simulink model "FORK"  (R2013b)
settings: Solver=ode45  StartTime=0.0  StopTime=2  RelTol=1e-3
libraries: powerlib x36, powerlib_meascontrol x6, powerlib_extras x3
settings Model: Creator=Yugal  LastModifiedBy=internship

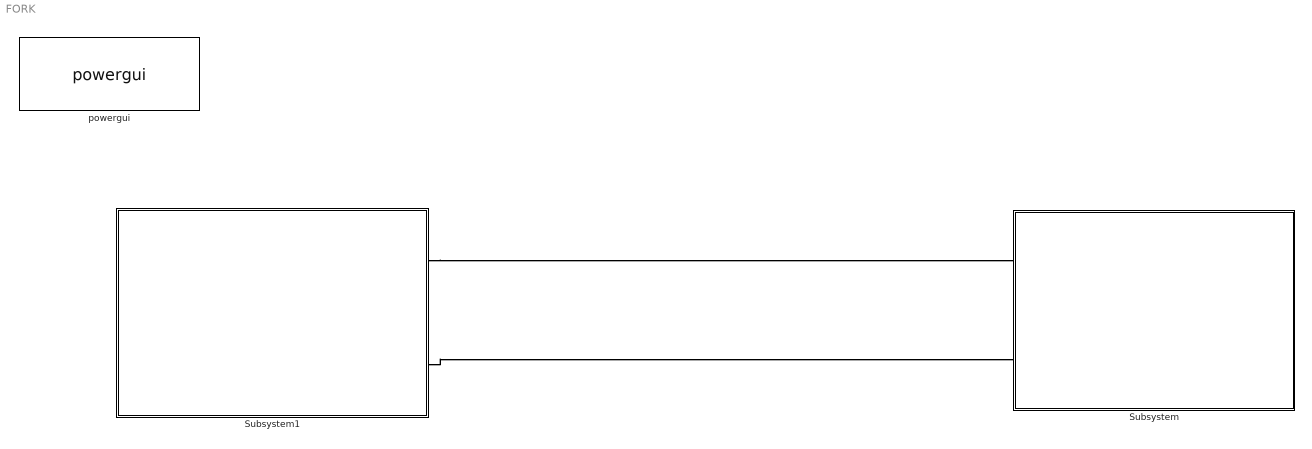
== system FORK ==
  Subsystem : Subsystem
  Subsystem1 : Subsystem
  powergui : powerlib/powergui  Priority=1  SimulationMode=Discrete  SolverType=Tustin  SampleTime=10e-6  frequency=60  SPID=off  DisableSnubberDevices=off  DisableRonSwitches=off  DisableVfSwitches=off  SwTol=0  Interpol=off  DisplayEquations=off  frequencyindice=50  Pbase=100e6  ErrMax=1e-4  Iterations=50  UnitsV=kV  UnitsW=MW  FunctionMessages=off  echomessages=off  HookPort=off  EnableUseOfTLC=off  x0status=blocks  RestoreLinks=warning  ResistiveCurrentMeasurement=off  Frange=[0:2:500]  Ylog=off  Xlog=on  ShowGrid=off  save=off  variable=ZData  structure=Ia  ZoomFFT=on  StartTime=1.5  cycles=2  DisplayStyle=1  fundamental=50  FreqAxis=on  MaxFrequency=1000  frequencyindicesteady=1  RmsSteady=1  display=off  Ts=100  methode=off
  connections:
  Subsystem1/RConn1 -- Subsystem/LConn1
  Subsystem1/RConn2 -- Subsystem/LConn2

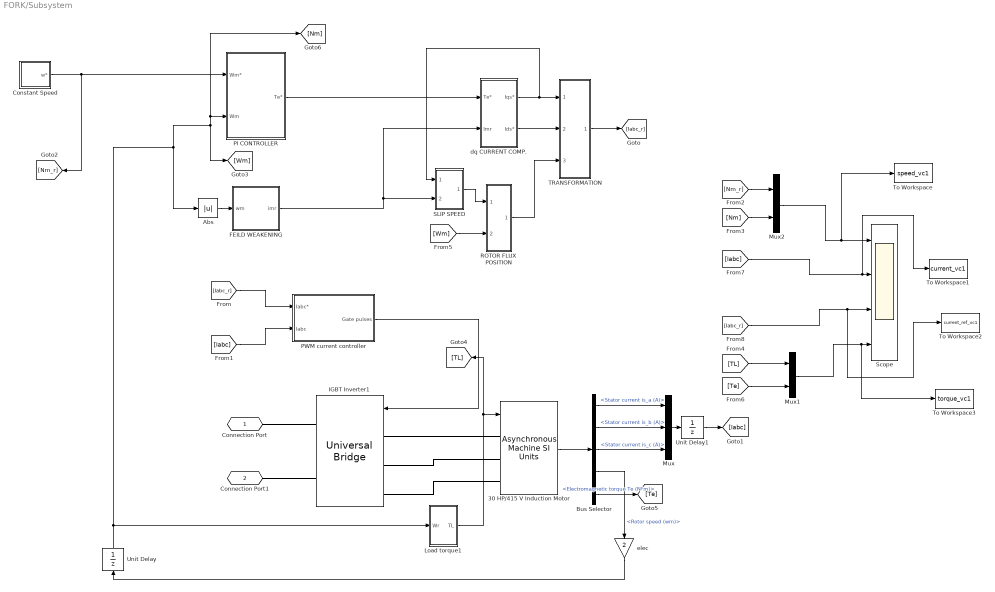
== system FORK/Subsystem ==
  30 HP/415 V Induction Motor : powerlib/Machines/Asynchronous Machine SI Units  PresetModel=No  MechanicalLoad=Torque Tm  ShowDetailedParameters=on  RotorType=Squirrel-cage  ReferenceFrame=Rotor  NominalParameters=[30*746 415 50]  Stator=[0.251 0.001397]  Rotor=[0.249 0.001397]  Cage1=[ 0.022 0.226/377]  Cage2=[ 0.022 0.226/377]  Lm=0.0416  Mechanical=[0.305 0 2 ]  PolePairs=2  InitialConditions=[1 0 0 0 0 0 0 0]  Units=SI  LoadFlowParameters=1492000  SimulateSaturation=off  Saturation=[14.03593122, 27.81365428, 53.79336849, 72.68890987, 97.98006896, 148.6815601, 215.7428561, 302.9841135, 420.4778367 ; 230, 322, 414, 460, 506, 552, 598, 644, 690]  TsPowergui=0  TsBlock=-1  IterativeModel=Trapezoidal non iterative  Pmec=0
  Abs : Abs  SaturateOnIntegerOverflow=on
  Bus Selector : BusSelector  OutputSignals=Stator measurements.Stator current is_a (A),Stator measurements.Stator current is_b (A),Stator measurements.Stator current is_c (A),Mechanical.Rotor speed (wm),Mechanical.Electromagnetic torque Te (N*m)
  Constant Speed : Subsystem
  FEILD WEAKENING : MATLAB Function  TreatAsAtomicUnit=on
  IGBT Inverter1 : powerlib/Power Electronics/Universal Bridge  Arms=3  SnubberResistance=1e5  SnubberCapacitance=inf  Device=MOSFET / Diodes  Ron=1e-3  Lon=0  ForwardVoltages="[  0  0  ]"  ForwardVoltage=0  GTOparameters=[ 10e-6 , 20e-6 ]  IGBTparameters=[ 1e-6 , 2e-6 ]  Measurements=None  Measurements_2=None  converterType=Rectifier
  Load torque1 : Subsystem
  Mux : Mux  Inputs=3
  Mux1 : Mux  Inputs=2
  Mux2 : Mux  Inputs=2
  PI CONTROLLER : Subsystem  mask{Kp=90, Ki=2.6, Ts=100e-6, Lim=300}
      mask prompts: Ts "Sampling Time Ts (sec)"; Lim "Ref Torque limit(N-m)"
  PWM current controller : Subsystem
  ROTOR FLUX POSITION : Subsystem
  SLIP SPEED : Subsystem
  Scope : Scope  NumInputPorts=4
      settings: TickLabels=on  TimeRange=4.5  YMin=249.989~-25~-22.5~-11  YMax=250.008~25~22.5~7  MaxDataPoints=1000  Decimation=10
  TRANSFORMATION : Subsystem
  To Workspace : ToWorkspace  VariableName=speed_vc1  SampleTime=100e-6  SaveFormat=Structure With Time
  To Workspace1 : ToWorkspace  VariableName=current_vc1  SampleTime=100e-6  SaveFormat=Structure With Time
  To Workspace2 : ToWorkspace  VariableName=current_ref_vc1  SampleTime=100e-6  SaveFormat=Structure With Time
  To Workspace3 : ToWorkspace  VariableName=torque_vc1  SampleTime=100e-6  SaveFormat=Structure With Time
  Unit Delay : UnitDelay  SampleTime=100e-6
  Unit Delay1 : UnitDelay  SampleTime=10e-6
  dq CURRENT COMP. : Subsystem
  elec : Gain  Gain=2
  Connection Port : PMIOPort  Port=1  Side=Left
  Connection Port1 : PMIOPort  Port=2  Side=Left
  wires:
  PWM current controller/1(Gate pulses) -> IGBT Inverter1/1
  Load torque1/1(TL) -> [TL], 30 HP/415 V Induction Motor/1
  30 HP/415 V Induction Motor/1 -> Bus Selector/1
  Bus Selector/3 -> Mux/3  "<Stator current is_c (A)>"
  Bus Selector/2 -> Mux/2  "<Stator current is_b (A)>"
  Bus Selector/1 -> Mux/1  "<Stator current is_a (A)>"
  [Iabc] -> PWM current controller/2(Iabc)
  [Iabc_r] -> PWM current controller/1(Iabc*)
  Abs/1 -> FEILD WEAKENING/1(wm)
  dq CURRENT COMP./2(Ids*) -> TRANSFORMATION/2(Ids*)
  dq CURRENT COMP./1(Iqs*) -> SLIP SPEED/1(Iqs*), TRANSFORMATION/1(Iqs*)
  PI CONTROLLER/1(Te*) -> dq CURRENT COMP./1(Te*)
  FEILD WEAKENING/1(imr) -> SLIP SPEED/2(Imr*), dq CURRENT COMP./2(Imr)
  SLIP SPEED/1(Wsl) -> ROTOR FLUX POSITION/1("Wsl\t")
  ROTOR FLUX POSITION/1(theta) -> TRANSFORMATION/3(theta)
  [Wm] -> ROTOR FLUX POSITION/2(Wm)
  TRANSFORMATION/1(Iabc*) -> [Iabc_r]
  Bus Selector/5 -> [Te]  "<Electromagnetic torque Te (N*m)>"
  [Te] -> Mux1/2
  [TL] -> Mux1/1
  Bus Selector/4 -> elec/1  "<Rotor speed (wm)>"
  Mux1/1 -> To Workspace3/1, Scope/4
  [Nm_r] -> Mux2/1
  [Nm] -> Mux2/2
  Mux2/1 -> To Workspace/1, Scope/1
  [Iabc] -> To Workspace1/1, Scope/2
  Constant Speed/1(w*) -> PI CONTROLLER/1(Wm*), [Nm_r]
  [Iabc_r] -> To Workspace2/1, Scope/3
  Mux/1 -> Unit Delay1/1
  Unit Delay1/1 -> [Iabc]
  elec/1 -> Unit Delay/1
  Unit Delay/1 -> Load torque1/1(Wr), [Nm], PI CONTROLLER/2(Wm), [Wm], Abs/1
  connections:
  30 HP/415 V Induction Motor/LConn1 -- IGBT Inverter1/LConn1
  30 HP/415 V Induction Motor/LConn3 -- IGBT Inverter1/LConn3
  30 HP/415 V Induction Motor/LConn2 -- IGBT Inverter1/LConn2
  Connection Port/RConn1 -- IGBT Inverter1/RConn1
  Connection Port1/RConn1 -- IGBT Inverter1/RConn2

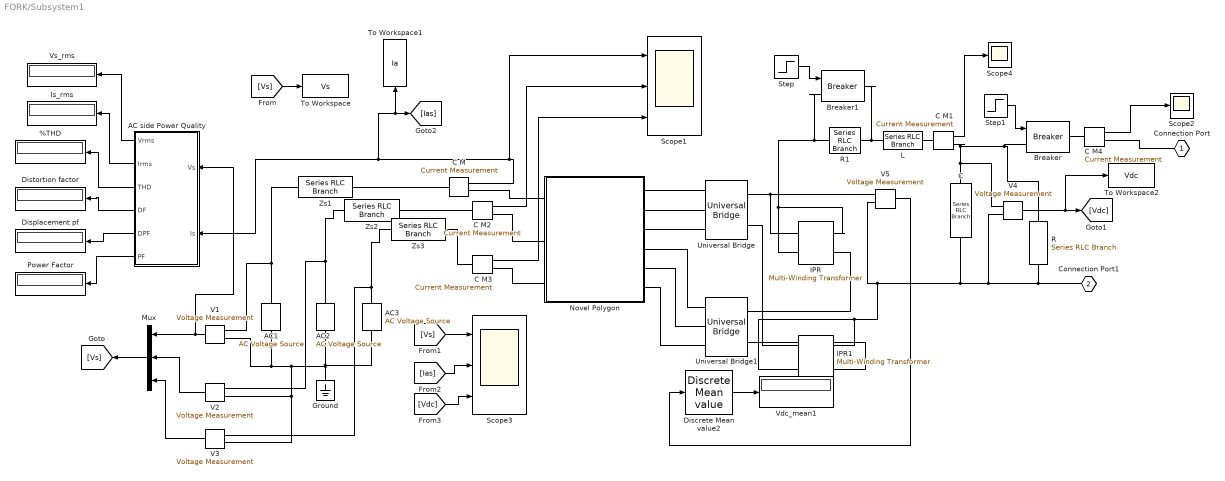
== system FORK/Subsystem1 ==
  %THD : Display
  AC side Power Quality : Subsystem
  AC1 : powerlib/Electrical Sources/AC Voltage Source  Amplitude=338.41  Phase=0  Frequency=50  SampleTime=0  Measurements=None
  AC2 : powerlib/Electrical Sources/AC Voltage Source  Amplitude=338.41  Phase=-120  Frequency=50  SampleTime=0  Measurements=None
  AC3 : powerlib/Electrical Sources/AC Voltage Source  Amplitude=338.41  Phase=-240  Frequency=50  SampleTime=0  Measurements=None
  Breaker : powerlib/Elements/Breaker  BreakerResistance=0.01  InitialState=0  SnubberResistance=1e6  SnubberCapacitance=inf  SwitchingTimes="[ 1/60  5/60 ]"  External=on  Measurements=None  MoreParameters=off  NoBreakLoop=off
  Breaker1 : powerlib/Elements/Breaker  BreakerResistance=0.01  InitialState=0  SnubberResistance=1e6  SnubberCapacitance=inf  SwitchingTimes="[ 1/60  5/60 ]"  External=on  Measurements=None  MoreParameters=off  NoBreakLoop=off
  "C " : powerlib/Elements/Series RLC Branch  LConnTagsString=__new0  RConnTagsString=__new0  BranchType=C  Resistance=1  Inductance=1e-3  SetiL0=off  InitialCurrent=0  Capacitance=1500e-6  Setx0=off  InitialVoltage=0  Measurements=Branch voltage
  C M{,1..4} (5 alike) : powerlib/Measurements/Current Measurement  PhasorSimulation=off  OutputType=Complex  PSBequivalent=0
  Discrete Mean value2 : powerlib_extras/Discrete Measurements/Discrete  Mean value  Freq=50  Vinit=0  Ts=5e-006
  Displacement pf : Display
  Distortion factor : Display
  Ground : powerlib/Elements/Ground  LConnTagsString=a
  IPR : powerlib/Elements/Multi-Winding Transformer  LeftWindings=1  RightWindings=1  TappedWindings=no taps  NumberOfTaps=2  UNITS=pu  NominalPower=[1.40e3 50]  NominalVoltages="[ 100  100 ]"  WindingResistances="[ 0.005  0.005 ]"  WindingInductances="[ 0.02  0.02 ]"  SetSaturation=off  Rm=50  Lm=50  Saturation=[ 0,0 ; 0.0024,1.2 ; 1.0,1.52 ]  Hysteresis=off  DataFile='hysteresis.mat'  Measurements=None  MoreParameters=off  BreakLoop=off  DataType=off  InitialFlux=0  TransfoNumber=1
  IPR1 : powerlib/Elements/Multi-Winding Transformer  LeftWindings=1  RightWindings=1  TappedWindings=no taps  NumberOfTaps=2  UNITS=pu  NominalPower=[1.40e3 50]  NominalVoltages="[ 100  100 ]"  WindingResistances="[ 0.005  0.005 ]"  WindingInductances="[ 0.02  0.02 ]"  SetSaturation=off  Rm=50  Lm=50  Saturation=[ 0,0 ; 0.0024,1.2 ; 1.0,1.52 ]  Hysteresis=off  DataFile='hysteresis.mat'  Measurements=None  MoreParameters=off  BreakLoop=off  DataType=off  InitialFlux=0  TransfoNumber=1
  Is_rms : Display
  L : powerlib/Elements/Series RLC Branch  LConnTagsString=__new0  RConnTagsString=__new0  BranchType=L  Resistance=1  Inductance=2e-3  SetiL0=off  InitialCurrent=0  Capacitance=1e-6  Setx0=off  InitialVoltage=0  Measurements=None
  Mux : Mux  Inputs=3
  Novel Polygon : Subsystem
  Power Factor : Display
  R : powerlib/Elements/Series RLC Branch  LConnTagsString=__new0  RConnTagsString=__new0  BranchType=R  Resistance=15  Inductance=1e-3  SetiL0=off  InitialCurrent=0  Capacitance=1e-6  Setx0=off  InitialVoltage=0  Measurements=None
  R1 : powerlib/Elements/Series RLC Branch  LConnTagsString=__new0  RConnTagsString=__new0  BranchType=R  Resistance=5  Inductance=1e-3  SetiL0=off  InitialCurrent=0  Capacitance=1e-6  Setx0=off  InitialVoltage=0  Measurements=None
  Scope1 : Scope  NumInputPorts=3
      settings: YMin=-5~-5~-5  YMax=5~5~5  SaveName=Source1
  Scope2 : Scope
      settings: YMin=0  YMax=50  Decimation=3
  Scope3 : Scope  NumInputPorts=3
      settings: TickLabels=on  ShowLegends=on  YMin=-5~-5~-5  YMax=5~5~5  SaveName=Source
  Scope4 : Scope
      settings: YMin=0  YMax=50  SaveName=ScopeData2  Decimation=3
  Step : Step  Time=0.02  SampleTime=0
  Step1 : Step  Time=0.2  SampleTime=0
  To Workspace : ToWorkspace  VariableName=Vs  SampleTime=100e-6  SaveFormat=Structure With Time
  To Workspace1 : ToWorkspace  VariableName=Ia  SampleTime=100e-6  SaveFormat=Structure With Time
  To Workspace2 : ToWorkspace  VariableName=Vdc  SampleTime=100e-6  SaveFormat=Structure With Time
  Universal Bridge : powerlib/Power Electronics/Universal Bridge  Arms=3  SnubberResistance=1e5  SnubberCapacitance=inf  Device=Diodes  Ron=1e-3  Lon=0  ForwardVoltages="[  0  0  ]"  ForwardVoltage=0  GTOparameters=[ 10e-6 , 20e-6 ]  IGBTparameters=[ 1e-6 , 2e-6 ]  Measurements=None  Measurements_2=None  converterType=Rectifier
  Universal Bridge1 : powerlib/Power Electronics/Universal Bridge  Arms=3  SnubberResistance=1e5  SnubberCapacitance=inf  Device=Diodes  Ron=1e-3  Lon=0  ForwardVoltages="[  0  0  ]"  ForwardVoltage=0  GTOparameters=[ 10e-6 , 20e-6 ]  IGBTparameters=[ 1e-6 , 2e-6 ]  Measurements=None  Measurements_2=None  converterType=Rectifier
  V{1..5} (5 alike) : powerlib/Measurements/Voltage Measurement  PhasorSimulation=off  OutputType=Complex  PSBequivalent=0
  Vdc_mean1 : Display
      settings: SampleTime=5e-006
  Vs_rms : Display
  Zs1 : powerlib/Elements/Series RLC Branch  LConnTagsString=__new0  RConnTagsString=__new0  BranchType=RL  Resistance=0.01  Inductance=1e-3  SetiL0=off  InitialCurrent=0  Capacitance=1e-6  Setx0=off  InitialVoltage=0  Measurements=None
  Zs2 : powerlib/Elements/Series RLC Branch  LConnTagsString=__new0  RConnTagsString=__new0  BranchType=RL  Resistance=0.01  Inductance=1e-3  SetiL0=off  InitialCurrent=0  Capacitance=1e-6  Setx0=off  InitialVoltage=0  Measurements=None
  Zs3 : powerlib/Elements/Series RLC Branch  LConnTagsString=__new0  RConnTagsString=__new0  BranchType=RL  Resistance=0.01  Inductance=1e-3  SetiL0=off  InitialCurrent=0  Capacitance=1e-6  Setx0=off  InitialVoltage=0  Measurements=None
  Connection Port : PMIOPort  Port=1  Side=Right
  Connection Port1 : PMIOPort  Port=2  Side=Right
  wires:
  V2/1 -> Mux/2
  V3/1 -> Mux/3
  Mux/1 -> [Vs]
  Step/1 -> Breaker1/1
  Step1/1 -> Breaker/1
  V1/1 -> AC side Power Quality/1(Vs), Mux/1
  V4/1 -> To Workspace2/1, [Vdc]
  C M1/1 -> Scope4/1
  V5/1 -> Discrete Mean value2/1
  Discrete Mean value2/1 -> Vdc_mean1/1
  C M4/1 -> Scope2/1
  AC side Power Quality/1("Vrms ") -> Vs_rms/1
  AC side Power Quality/2(Irms) -> Is_rms/1
  AC side Power Quality/3("THD ") -> %THD/1
  AC side Power Quality/4(DF) -> Distortion factor/1
  AC side Power Quality/5(DPF) -> Displacement pf/1
  AC side Power Quality/6(PF) -> Power Factor/1
  C M2/1 -> Scope1/2
  C M3/1 -> Scope1/3
  [Vs] -> To Workspace/1
  C M/1 -> Scope1/1, To Workspace1/1, [Ias], AC side Power Quality/2(Is)
  [Vs] -> Scope3/1
  [Ias] -> Scope3/2
  [Vdc] -> Scope3/3
  connections:
  AC1/LConn1 -- V1/LConn2 -- V3/LConn2 -- V2/LConn2 -- Ground/LConn1 -- AC3/LConn1 -- AC2/LConn1
  Breaker/LConn1 -- R/LConn1 -- C M1/RConn1 -- "C "/LConn1 -- V4/LConn1
  L/LConn1 -- Breaker1/RConn1 -- R1/RConn1
  "C "/RConn1 -- IPR1/RConn1 -- IPR1/LConn2 -- V5/LConn2 -- V4/LConn2 -- Connection Port1/RConn1 -- R/RConn1
  AC1/RConn1 -- Zs1/LConn1 -- V1/LConn1
  V2/LConn1 -- Zs2/LConn1 -- AC2/RConn1
  V3/LConn1 -- Zs3/LConn1 -- AC3/RConn1
  Universal Bridge/RConn1 -- V5/LConn1 -- IPR/LConn1
  R1/LConn1 -- Breaker1/LConn1 -- IPR/LConn2 -- IPR/RConn1
  Zs3/RConn1 -- C M3/LConn1
  Universal Bridge1/RConn1 -- IPR/RConn2
  Zs1/RConn1 -- C M/LConn1
  Zs2/RConn1 -- C M2/LConn1
  Breaker/RConn1 -- C M4/LConn1
  L/RConn1 -- C M1/LConn1
  Novel Polygon/LConn1 -- C M/RConn1
  C M4/RConn1 -- Connection Port/RConn1
  C M2/RConn1 -- Novel Polygon/LConn2
  C M3/RConn1 -- Novel Polygon/LConn3
  Universal Bridge/LConn1 -- Novel Polygon/RConn1
  Universal Bridge/LConn2 -- Novel Polygon/RConn2
  Universal Bridge/LConn3 -- Novel Polygon/RConn3
  Universal Bridge1/LConn1 -- Novel Polygon/RConn4
  Universal Bridge1/LConn2 -- Novel Polygon/RConn5
  Universal Bridge1/LConn3 -- Novel Polygon/RConn6
  Universal Bridge/RConn2 -- IPR1/LConn1
  IPR1/RConn2 -- Universal Bridge1/RConn2

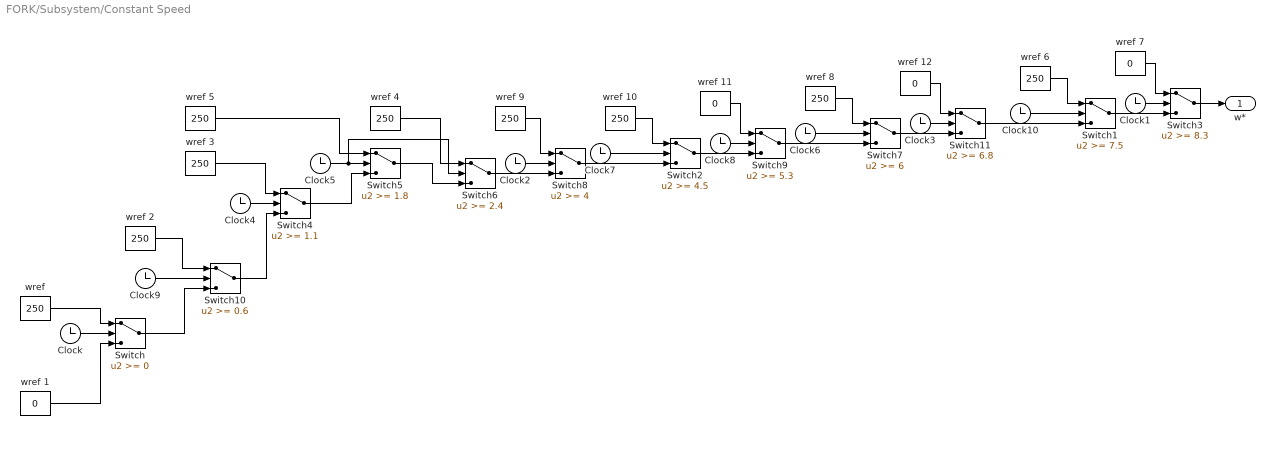
== system FORK/Subsystem/Constant Speed ==
  Clock{,1..10} (11 alike) : Clock
      settings: Decimation=2
  Switch : Switch  SaturateOnIntegerOverflow=on  InputSameDT=on
  Switch1 : Switch  Threshold=7.5  SaturateOnIntegerOverflow=on  InputSameDT=on
  Switch10 : Switch  Threshold=0.6  SaturateOnIntegerOverflow=on  InputSameDT=on
  Switch11 : Switch  Threshold=6.8  SaturateOnIntegerOverflow=on  InputSameDT=on
  Switch2 : Switch  Threshold=4.5  SaturateOnIntegerOverflow=on  InputSameDT=on
  Switch3 : Switch  Threshold=8.3  SaturateOnIntegerOverflow=on  InputSameDT=on
  Switch4 : Switch  Threshold=1.1  SaturateOnIntegerOverflow=on  InputSameDT=on
  Switch5 : Switch  Threshold=1.8  SaturateOnIntegerOverflow=on  InputSameDT=on
  Switch6 : Switch  Threshold=2.4  SaturateOnIntegerOverflow=on  InputSameDT=on
  Switch7 : Switch  Threshold=6  SaturateOnIntegerOverflow=on  InputSameDT=on
  Switch8 : Switch  Threshold=4  SaturateOnIntegerOverflow=on  InputSameDT=on
  Switch9 : Switch  Threshold=5.3  SaturateOnIntegerOverflow=on  InputSameDT=on
  wref {,2..6,8..10} (9 alike) : Constant  Value=250
  wref {1,7,11..12} (4 alike) : Constant  Value=0
  w* : Outport
  wires:
  wref 1/1 -> Switch/3
  Clock/1 -> Switch/2
  "wref "/1 -> Switch/1
  Clock4/1 -> Switch4/2
  wref 3/1 -> Switch4/1
  Switch4/1 -> Switch5/3
  Switch5/1 -> Switch6/3
  Clock5/1 -> Switch6/2, Switch5/2
  wref 4/1 -> Switch6/1
  wref 5/1 -> Switch5/1
  Switch10/1 -> Switch4/3
  Switch6/1 -> Switch8/3
  wref 9/1 -> Switch8/1
  Clock2/1 -> Switch8/2
  Switch8/1 -> Switch2/3
  Clock7/1 -> Switch2/2
  wref 10/1 -> Switch2/1
  Switch2/1 -> Switch9/3
  Clock8/1 -> Switch9/2
  wref 11/1 -> Switch9/1
  Switch/1 -> Switch10/3
  Clock9/1 -> Switch10/2
  wref 2/1 -> Switch10/1
  Switch11/1 -> Switch1/3
  Clock10/1 -> Switch1/2
  wref 6/1 -> Switch1/1
  Switch1/1 -> Switch3/3
  Clock1/1 -> Switch3/2
  wref 7/1 -> Switch3/1
  Clock6/1 -> Switch7/2
  wref 8/1 -> Switch7/1
  Switch7/1 -> Switch11/3
  Clock3/1 -> Switch11/2
  wref 12/1 -> Switch11/1
  Switch9/1 -> Switch7/3
  Switch3/1 -> w*/1

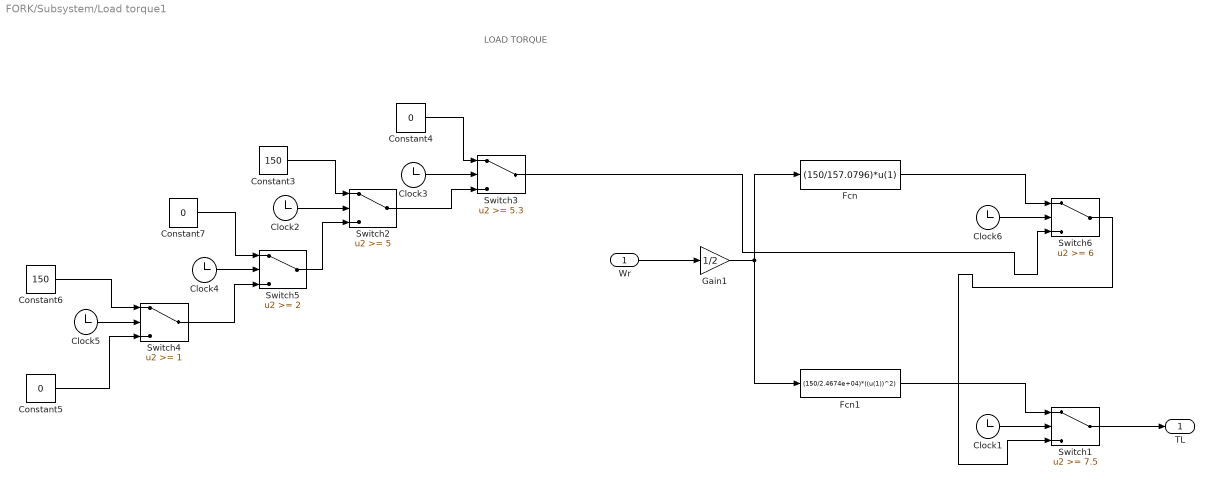
== system FORK/Subsystem/Load torque1 ==
  note: LOAD TORQUE
  Wr : Inport
  Clock{1..6} (6 alike) : Clock
  Constant3 : Constant  Value=150
  Constant4 : Constant  Value=0
  Constant5 : Constant  Value=0
  Constant6 : Constant  Value=150
  Constant7 : Constant  Value=0
  Fcn : Fcn  Expr=(150/157.0796)*u(1)
  Fcn1 : Fcn  Expr=(150/2.4674e+04)*((u(1))^2)
  Gain1 : Gain  Gain=1/2
  Switch1 : Switch  Threshold=7.5
  Switch2 : Switch  Threshold=5
  Switch3 : Switch  Threshold=5.3
  Switch4 : Switch  Threshold=1
  Switch5 : Switch  Threshold=2
  Switch6 : Switch  Threshold=6
  TL : Outport
  wires:
  Switch5/1 -> Switch2/3
  Clock2/1 -> Switch2/2
  Switch2/1 -> Switch3/3
  Clock3/1 -> Switch3/2
  Constant3/1 -> Switch2/1
  Constant4/1 -> Switch3/1
  Wr/1 -> Gain1/1
  Gain1/1 -> Fcn/1, Fcn1/1
  Constant5/1 -> Switch4/3
  Constant6/1 -> Switch4/1
  Switch4/1 -> Switch5/3
  Clock4/1 -> Switch5/2
  Constant7/1 -> Switch5/1
  Clock5/1 -> Switch4/2
  Clock6/1 -> Switch6/2
  Fcn/1 -> Switch6/1
  Switch3/1 -> Switch6/3
  Clock1/1 -> Switch1/2
  Fcn1/1 -> Switch1/1
  Switch6/1 -> Switch1/3
  Switch1/1 -> TL/1

== system FORK/Subsystem/PI CONTROLLER ==
  note: Wm*
  note: Wm
  Wm* : Inport
  Wm : Inport  Port=2
  Subsystem : Subsystem
  Sum : Sum  Inputs=|+-
  Te* : Outport
  wires:
  Wm*/1 -> Sum/1
  Subsystem/1(Te*) -> Te*/1
  Sum/1 -> Subsystem/1(We)
  Wm/1 -> Sum/2

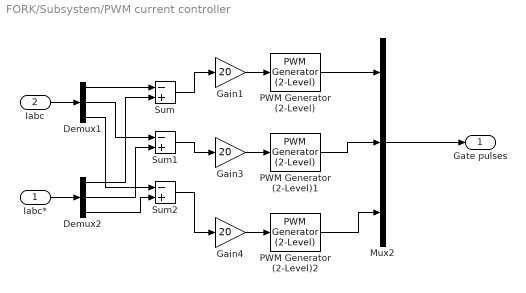
== system FORK/Subsystem/PWM current controller ==
  Iabc* : Inport
  Iabc : Inport  Port=2
  Demux1 : Demux  Outputs=3
  Demux2 : Demux  Outputs=3
  Gain1 : Gain  Gain=20  SaturateOnIntegerOverflow=on  OutDataTypeStr=Inherit: Same as input  ParamDataTypeStr=Inherit: Same as input
  Gain3 : Gain  Gain=20  SaturateOnIntegerOverflow=on  OutDataTypeStr=Inherit: Same as input  ParamDataTypeStr=Inherit: Same as input
  Gain4 : Gain  Gain=20  SaturateOnIntegerOverflow=on  OutDataTypeStr=Inherit: Same as input  ParamDataTypeStr=Inherit: Same as input
  Mux2 : Mux  Inputs=3
  PWM Generator (2-Level) : powerlib_meascontrol/Pulse & Signal Generators/PWM Generator (2-Level)  ModulatorType=Single-phase half-bridge (2 pulses)  ModulatorMode=Unsynchronized  nF=27  Fc=10000  ModulatingSignals=off  m=0.8  Freq=60  Phase=0  Ts=10e-6
  PWM Generator (2-Level)1 : powerlib_meascontrol/Pulse & Signal Generators/PWM Generator (2-Level)  ModulatorType=Single-phase half-bridge (2 pulses)  ModulatorMode=Unsynchronized  nF=27  Fc=10000  ModulatingSignals=off  m=0.8  Freq=60  Phase=0  Ts=5e-6
  PWM Generator (2-Level)2 : powerlib_meascontrol/Pulse & Signal Generators/PWM Generator (2-Level)  ModulatorType=Single-phase half-bridge (2 pulses)  ModulatorMode=Unsynchronized  nF=27  Fc=10000  ModulatingSignals=off  m=0.8  Freq=60  Phase=0  Ts=5e-6
  Sum : Sum  Inputs=-+  SaturateOnIntegerOverflow=on  InputSameDT=on  OutDataTypeStr=Inherit: Same as first input
  Sum1 : Sum  Inputs=-+  SaturateOnIntegerOverflow=on  InputSameDT=on  OutDataTypeStr=Inherit: Same as first input
  Sum2 : Sum  Inputs=-+  SaturateOnIntegerOverflow=on  InputSameDT=on  OutDataTypeStr=Inherit: Same as first input
  Gate pulses : Outport
  wires:
  PWM Generator (2-Level)/1 -> Mux2/1
  PWM Generator (2-Level)1/1 -> Mux2/2
  PWM Generator (2-Level)2/1 -> Mux2/3
  Gain3/1 -> PWM Generator (2-Level)1/1
  Gain4/1 -> PWM Generator (2-Level)2/1
  Mux2/1 -> Gate pulses/1
  Gain1/1 -> PWM Generator (2-Level)/1
  Demux1/1 -> Sum/1
  Demux1/2 -> Sum1/1
  Iabc/1 -> Demux1/1
  Demux1/3 -> Sum2/1
  Demux2/3 -> Sum2/2
  Demux2/2 -> Sum1/2
  Demux2/1 -> Sum/2
  Iabc*/1 -> Demux2/1
  Sum/1 -> Gain1/1
  Sum1/1 -> Gain3/1
  Sum2/1 -> Gain4/1

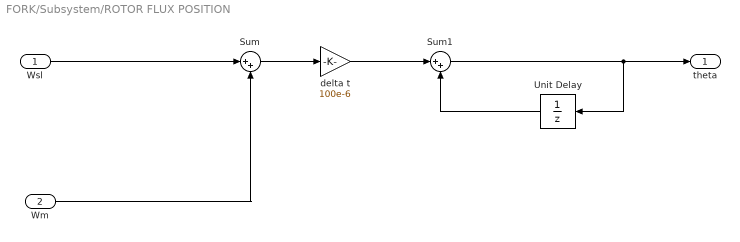
== system FORK/Subsystem/ROTOR FLUX POSITION ==
  "Wsl\t" : Inport
  Wm : Inport  Port=2
  Sum : Sum  Inputs=|++
  Sum1 : Sum  Inputs=|++
  Unit Delay : UnitDelay  SampleTime=100e-6
  delta t : Gain  Gain=100e-6
  theta : Outport
  wires:
  delta t/1 -> Sum1/1
  Sum1/1 -> Unit Delay/1, theta/1
  Sum/1 -> delta t/1
  Unit Delay/1 -> Sum1/2
  Wm/1 -> Sum/2
  "Wsl\t"/1 -> Sum/1

== system FORK/Subsystem/SLIP SPEED ==
  Iqs* : Inport
  Imr* : Inport  Port=2
  Gain : Gain  Gain=0.17296
  Product : Product  Inputs=*/
  Wsl : Outport
  wires:
  Iqs*/1 -> Product/1
  Product/1 -> Wsl/1
  Gain/1 -> Product/2
  Imr*/1 -> Gain/1

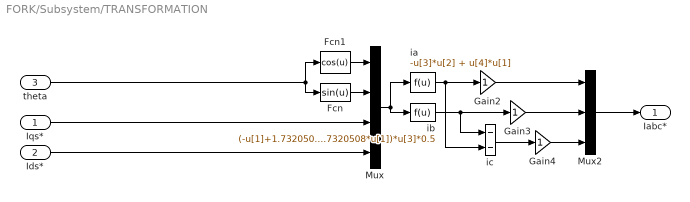
== system FORK/Subsystem/TRANSFORMATION ==
  Iqs* : Inport
  Ids* : Inport  Port=2
  theta : Inport  Port=3
  Fcn : Fcn  Expr=sin(u)
  Fcn1 : Fcn  Expr=cos(u)
  Gain2 : Gain  SaturateOnIntegerOverflow=on  OutDataTypeStr=Inherit: Same as input  ParamDataTypeStr=Inherit: Same as input
  Gain3 : Gain  SaturateOnIntegerOverflow=on  OutDataTypeStr=Inherit: Same as input  ParamDataTypeStr=Inherit: Same as input
  Gain4 : Gain  SaturateOnIntegerOverflow=on  OutDataTypeStr=Inherit: Same as input  ParamDataTypeStr=Inherit: Same as input
  Mux : Mux
  Mux2 : Mux  Inputs=3
  ia : Fcn  Expr=-u[3]*u[2] + u[4]*u[1]
  ib : Fcn  Expr=(-u[1]+1.7320508*u[2])*u[4]*0.5+(u[2]+1.7320508*u[1])*u[3]*0.5
  ic : Sum  Inputs=--  SaturateOnIntegerOverflow=on  InputSameDT=on  OutDataTypeStr=Inherit: Same as first input
  Iabc* : Outport
  wires:
  Fcn/1 -> Mux/2
  theta/1 -> Fcn/1, Fcn1/1
  Mux2/1 -> Iabc*/1
  Gain3/1 -> Mux2/2
  Fcn1/1 -> Mux/1
  ic/1 -> Gain4/1
  ib/1 -> Gain3/1, ic/1
  Mux/1 -> ib/1, ia/1
  ia/1 -> Gain2/1, ic/2
  Iqs*/1 -> Mux/3
  Ids*/1 -> Mux/4
  Gain2/1 -> Mux2/1
  Gain4/1 -> Mux2/3

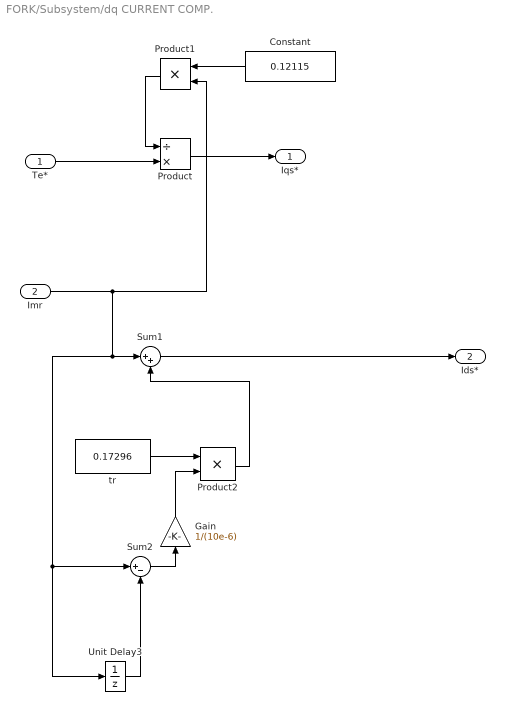
== system FORK/Subsystem/dq CURRENT COMP. ==
  Te* : Inport
  Imr : Inport  Port=2
  Constant : Constant  Value=0.12115
  Gain : Gain  Gain=1/(10e-6)
  Product : Product  Inputs=/*
  Product1 : Product
  Product2 : Product  SaturateOnIntegerOverflow=on  InputSameDT=on  OutDataTypeStr=Inherit: Same as first input
  Sum1 : Sum  Inputs=|++
  Sum2 : Sum  Inputs=|+-
  Unit Delay3 : UnitDelay  SampleTime=10e-6
  tr : Constant  Value=0.17296
  Iqs* : Outport
  Ids* : Outport  Port=2
  wires:
  Product1/1 -> Product/1
  Constant/1 -> Product1/1
  Te*/1 -> Product/2
  Product/1 -> Iqs*/1
  Imr/1 -> Sum2/1, Unit Delay3/1, Sum1/1, Product1/2
  tr/1 -> Product2/1
  Product2/1 -> Sum1/2
  Sum1/1 -> Ids*/1
  Unit Delay3/1 -> Sum2/2
  Sum2/1 -> Gain/1
  Gain/1 -> Product2/2

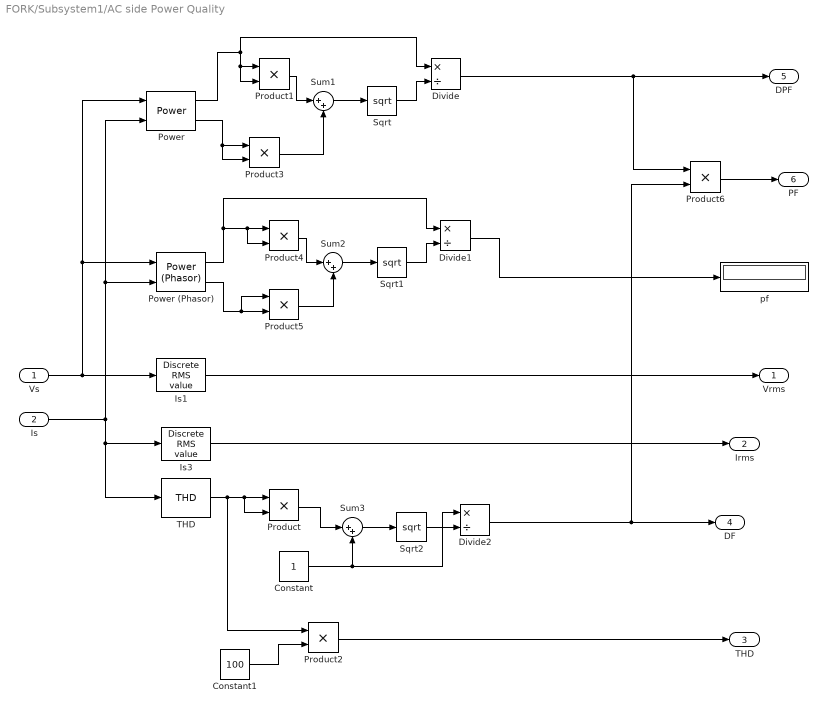
== system FORK/Subsystem1/AC side Power Quality ==
  Vs : Inport
  Is : Inport  Port=2
  Constant : Constant
  Constant1 : Constant  Value=100
  Divide : Product  Inputs=*/
  Divide1 : Product  Inputs=*/
  Divide2 : Product  Inputs=*/
  Is1 : powerlib_extras/Discrete Measurements/Discrete  RMS value  Freq=50  Mag_Init=0  Ts=5e-006
  Is3 : powerlib_extras/Discrete Measurements/Discrete  RMS value  Freq=50  Mag_Init=0  Ts=5e-006
  Power : powerlib_meascontrol/Measurements/Power  Freq=60  Vinit=[1, 0]  Iinit=[1, 0]  Ts=0
  Power (Phasor) : powerlib_meascontrol/Measurements/Power (Phasor)
  Product{,1..6} (7 alike) : Product
  Sqrt : Sqrt  SaturateOnIntegerOverflow=on
  Sqrt1 : Sqrt  SaturateOnIntegerOverflow=on
  Sqrt2 : Sqrt  SaturateOnIntegerOverflow=on
  Sum1 : Sum  Inputs=|++
  Sum2 : Sum  Inputs=|++
  Sum3 : Sum  Inputs=|++
  THD : powerlib_meascontrol/Measurements/THD  Freq=50  Ts=5e-006
  pf : Display
  "Vrms " : Outport
  Irms : Outport  Port=2
  "THD " : Outport  Port=3
  DF : Outport  Port=4
  DPF : Outport  Port=5
  PF : Outport  Port=6
  wires:
  Vs/1 -> Is1/1, Power/1, Power (Phasor)/1
  Is/1 -> Power/2, Power (Phasor)/2, Is3/1, THD/1
  Power/1 -> Product1/2, Product1/1, Divide/1
  Power/2 -> Product3/1, Product3/2
  Product1/1 -> Sum1/1
  Product3/1 -> Sum1/2
  Sum1/1 -> Sqrt/1
  Sqrt/1 -> Divide/2
  Power (Phasor)/2 -> Product5/1, Product5/2
  Product4/1 -> Sum2/1
  Product5/1 -> Sum2/2
  Sum2/1 -> Sqrt1/1
  Sqrt1/1 -> Divide1/2
  Divide1/1 -> pf/1
  THD/1 -> Product2/1, Product/2, Product/1
  Power (Phasor)/1 -> Product4/2, Product4/1, Divide1/1
  Product/1 -> Sum3/1
  Constant/1 -> Divide2/1, Sum3/2
  Sum3/1 -> Sqrt2/1
  Sqrt2/1 -> Divide2/2
  Divide2/1 -> DF/1, Product6/2
  Divide/1 -> Product6/1, DPF/1
  Constant1/1 -> Product2/2
  Is1/1 -> "Vrms "/1
  Is3/1 -> Irms/1
  Product2/1 -> "THD "/1
  Product6/1 -> PF/1

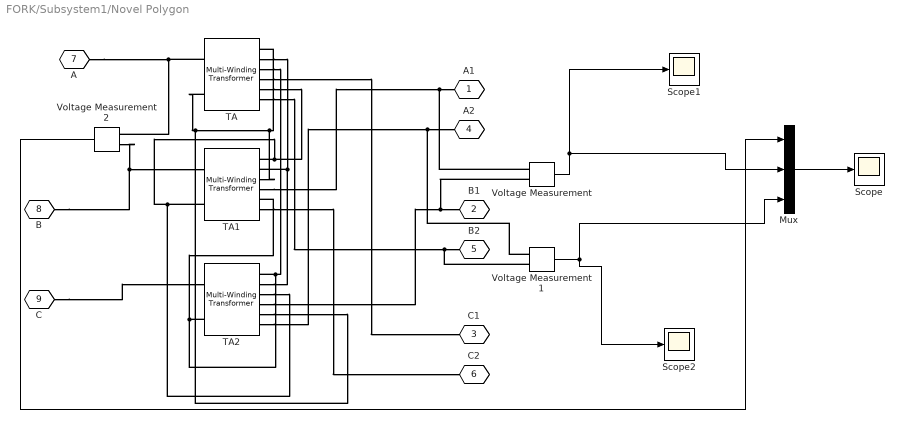
== system FORK/Subsystem1/Novel Polygon ==
  Mux : Mux  Inputs=3
  Scope : Scope
      settings: YMin=-50  YMax=50  SaveName=ScopeData5
  Scope1 : Scope
      settings: YMin=-1000  YMax=1000  SaveName=star
  Scope2 : Scope
      settings: YMin=-1000  YMax=1000  SaveName=delta
  TA : powerlib/Elements/Multi-Winding Transformer  LeftWindings=1  RightWindings=3  TappedWindings=no taps  NumberOfTaps=2  UNITS=pu  NominalPower=[2.096e3 50]  NominalVoltages=[ 43.915 195.4047 71.5088 71.5088 ]  WindingResistances=[ 0.002 0.002 0.002 0.002]  WindingInductances=[ .08 .08 .08 .08 ]  SetSaturation=off  Rm=50  Lm=50  Saturation=[ 0,0 ; 0.0024,1.2 ; 1.0,1.52 ]  Hysteresis=off  DataFile='hysteresis.mat'  Measurements=None  MoreParameters=off  BreakLoop=off  DataType=off  InitialFlux=0  TransfoNumber=1
  TA1 : powerlib/Elements/Multi-Winding Transformer  LeftWindings=1  RightWindings=3  TappedWindings=no taps  NumberOfTaps=2  UNITS=pu  NominalPower=[2.096e3 50]  NominalVoltages=[ 43.915 195.4047 71.5088 71.5088 ]  WindingResistances=[ 0.002 0.002 .002 .002]  WindingInductances=[ .08 .08 .08 .08 ]  SetSaturation=off  Rm=50  Lm=50  Saturation=[ 0,0 ; 0.0024,1.2 ; 1.0,1.52 ]  Hysteresis=off  DataFile='hysteresis.mat'  Measurements=None  MoreParameters=off  BreakLoop=off  DataType=off  InitialFlux=0  TransfoNumber=1
  TA2 : powerlib/Elements/Multi-Winding Transformer  LeftWindings=1  RightWindings=3  TappedWindings=no taps  NumberOfTaps=2  UNITS=pu  NominalPower=[2.096e3 50]  NominalVoltages=[ 43.915 195.4047 71.5088 71.5088 ]  WindingResistances=[ 0.002 0.002 .002 .002]  WindingInductances="[  .08 .08 .08 .08 ]"  SetSaturation=off  Rm=50  Lm=50  Saturation=[ 0,0 ; 0.0024,1.2 ; 1.0,1.52 ]  Hysteresis=off  DataFile='hysteresis.mat'  Measurements=None  MoreParameters=off  BreakLoop=off  DataType=off  InitialFlux=0  TransfoNumber=1
  Voltage Measurement : powerlib/Measurements/Voltage Measurement  PhasorSimulation=off  OutputType=Complex  PSBequivalent=0
  Voltage Measurement1 : powerlib/Measurements/Voltage Measurement  PhasorSimulation=off  OutputType=Complex  PSBequivalent=0
  Voltage Measurement2 : powerlib/Measurements/Voltage Measurement  PhasorSimulation=off  OutputType=Complex  PSBequivalent=0
  A1 : PMIOPort  Tag=PMCPort  Port=1  Side=Right
  B1 : PMIOPort  Tag=PMCPort  Port=2  Side=Right
  C1 : PMIOPort  Tag=PMCPort  Port=3  Side=Right
  A2 : PMIOPort  Tag=PMCPort  Port=4  Side=Right
  B2 : PMIOPort  Tag=PMCPort  Port=5  Side=Right
  C2 : PMIOPort  Tag=PMCPort  Port=6  Side=Right
  A : PMIOPort  Tag=PMCPort  Port=7  Side=Left
  B : PMIOPort  Tag=PMCPort  Port=8  Side=Left
  C : PMIOPort  Tag=PMCPort  Port=9  Side=Left
  wires:
  Voltage Measurement2/1 -> Mux/1
  Voltage Measurement/1 -> Scope1/1, Mux/2
  Voltage Measurement1/1 -> Scope2/1, Mux/3
  Mux/1 -> Scope/1
  connections:
  A/RConn1 -- Voltage Measurement2/LConn1 -- TA/LConn1
  TA/LConn2 -- TA2/RConn5 -- TA1/RConn3 -- TA/RConn1
  TA/RConn2 -- TA2/RConn2 -- TA1/RConn2
  TA/RConn4 -- C1/RConn1
  TA/RConn5 -- TA2/RConn3 -- TA1/LConn2 -- TA1/RConn1
  TA/RConn6 -- Voltage Measurement1/LConn2 -- B2/RConn1
  B/RConn1 -- Voltage Measurement2/LConn2 -- TA1/LConn1
  TA1/RConn4 -- Voltage Measurement/LConn1 -- A1/RConn1
  TA/RConn3 -- TA1/RConn5 -- TA2/LConn2 -- TA2/RConn1
  TA1/RConn6 -- C2/RConn1
  C/RConn1 -- TA2/LConn1
  TA2/RConn4 -- Voltage Measurement/LConn2 -- B1/RConn1
  TA2/RConn6 -- Voltage Measurement1/LConn1 -- A2/RConn1

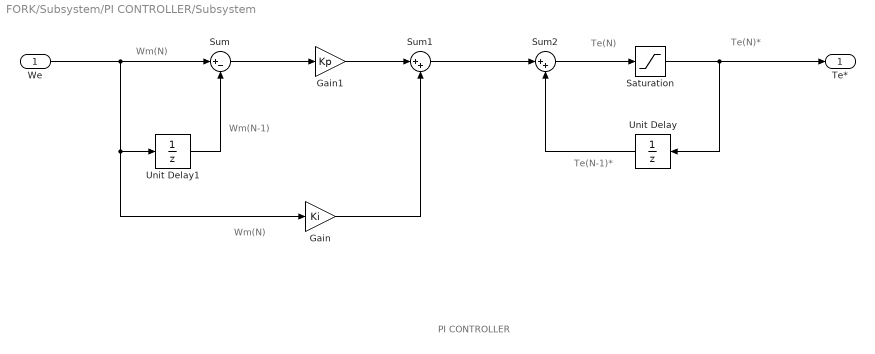
== system FORK/Subsystem/PI CONTROLLER/Subsystem ==
  note: PI CONTROLLER
  note: Wm(N)
  note: Wm(N-1)
  note: Wm(N)
  note: Te(N)
  note: Te(N)*
  note: Te(N-1)*
  We : Inport
  Gain : Gain  Gain=Ki
  Gain1 : Gain  Gain=Kp
  Saturation : Saturate  UpperLimit=Lim  LowerLimit=-Lim
  Sum : Sum  Inputs=|+-
  Sum1 : Sum  Inputs=|++
  Sum2 : Sum  Inputs=|++
  Unit Delay : UnitDelay  SampleTime=Ts
  Unit Delay1 : UnitDelay  SampleTime=Ts
  Te* : Outport
  wires:
  Sum1/1 -> Sum2/1
  Sum2/1 -> Saturation/1
  Saturation/1 -> Unit Delay/1, Te*/1
  Sum/1 -> Gain1/1
  Gain1/1 -> Sum1/1
  Unit Delay1/1 -> Sum/2
  We/1 -> Sum/1, Unit Delay1/1, Gain/1
  Gain/1 -> Sum1/2
  Unit Delay/1 -> Sum2/2

== matlab function FORK/Subsystem/FEILD WEAKENING ==
  data: wm input; imr output
function imr = fcn(wm)
%#codegen
if wm<2*pi*50
    imr=21.6;
else
    imr=2*pi*50*21.6/wm;
end
